simulink model "rpi_i2c_send"  (R2014a)
settings: Solver=FixedStepDiscrete  StartTime=0.0  StopTime=inf  RelTol=1e-3
libraries: embdlinuxlib x3, dspindex x2, visionstatistics x1, visiontextngfix x1, visionanalysis x1
settings Model: SimulationMode=external  ExtModeTrigDuration=100  Creator=mbelge  LastModifiedBy=planger
settings DataIOCC: SignalLoggingSaveFormat=ModelDataLogs
settings OptimizationCC: ExpressionDepthLimit=2147483647  OptimizeModelRefInitCode=on  LifeSpan=1
settings DebuggingCC: UnderspecifiedInitializationDetection=Classic  SolverPrmCheckMsg=none  FcnCallInpInsideContextMsg=EnableAllAsWarning  StateNameClashWarn=warning
settings HardwareCC: ProdLargestAtomicInteger=Long  ProdLargestAtomicFloat=Double  ProdEndianess=LittleEndian  ProdHWDeviceType=ARM Compatible->ARM Cortex
settings RTWCC: SystemTargetFile=realtime.tlc  GenerateMakefile=off  TemplateMakefile=realtime.tmf  Description=Real-Time Toolbox  RTWVerbose=off  ProcessScript=realtime_make_rtw_hook
settings CodeAppCC: CustomSymbolStrType=$N$R$M  InternalIdentifier=Classic
settings STFCustomTargetCC: TargetLibSuffix=.a  GenerateSampleERTMain=on  ConcurrentExecutionCompliant=off  GeneratePreprocessorConditionals=Use local settings  ERTCustomFileBanners=on  SupportNonInlinedSFcns=off  SupportVariableSizeSignals=on  MATLABClassNameForMDSCustomization=Simulink.SoftwareTarget.ERTCustomization  GRTInterface=off  SystemTargetFile=realtime.tlc
settings ERTTargetCC: CombineOutputUpdateFcns=off  SupportContinuousTime=on  SupportVariableSizeSignals=on  ExtMode=on  ExtModeMexArgs='plpi-wifi' 0 17725  ERTSrcFileBannerTemplate=realtime_code_template.cgt  ERTHdrFileBannerTemplate=realtime_code_template.cgt  ERTDataSrcFileTemplate=realtime_code_template.cgt  ERTDataHdrFileTemplate=realtime_code_template.cgt  ERTCustomFileTemplate=realtime_file_process.tlc

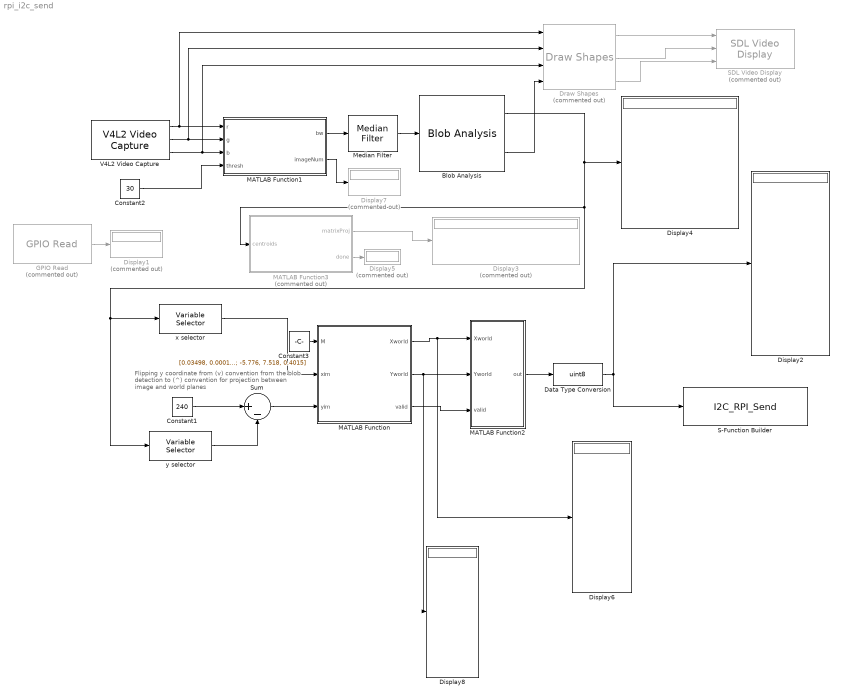
== system rpi_i2c_send ==
  note: Flipping y coordinate from (v) convention from
      | the blob detection to (^) convention for projection
      | between image and world planes
  Blob Analysis : visionstatistics/Blob Analysis  Tag=vipblks_row_conv  area=off  centroid=on  bBox=on  majorAxis=off  minorAxis=off  angle=off  eccentricity=off  equivDiameterSq=off  extent=off  perimeter=off  maxBlobs=6  warnIfNumBlobsExceeded=off  isCount=off  useMinArea=on  minArea=25  useMaxArea=off  maxArea=intmax('uint32')  excludeBorderBlob=on  outDT=single  isOutVarDim=off  isFill=on  fillValues=-1  conn=8  isLabel=off  outputMode=Binary point scaling  outputWordLength=32  outputFracLength=16  firstCoeffMode=Binary point scaling  firstCoeffWordLength=16  firstCoeffFracLength=14  secondCoeffMode=Binary point scaling  secondCoeffWordLength=32  secondCoeffFracLength=16  accumMode=Binary point scaling  accumWordLength=32  accumFracLength=0  prodOutputMode=Binary point scaling  prodOutputWordLength=32  prodOutputFracLength=16  roundingMode=Floor  overflowMode=off
  Constant1 : Constant  Value=240  OutDataTypeStr=single
  Constant2 : Constant  Value=30  OutDataTypeStr=single
  Constant3 : Constant  Value=[0.03498, 0.0001508, -4.339e-5; 0.001215, 0.01909, -0.001534; -5.776, 7.518, 0.4015]  VectorParams1D=off  OutDataTypeStr=single
  Data Type Conversion : DataTypeConversion  OutDataTypeStr=uint8
  Display{1,3,5,7} (4 alike) : Display  Commented=on
  Display{2,4,6,8} (4 alike) : Display
  Draw Shapes : visiontextngfix/Draw Shapes  Commented=on  shape=Rectangles  fill=off  lineWidth=1  fillClrSource=Specify via dialog  display=User-specified value  intensity=200  color=[0 0 0]  opacity=0.6  viewport=Entire image  antialiasing=off  inType=Obsolete  imagePorts=Separate color signals  prodOutputMode=Binary point scaling  prodOutputWordLength=32  prodOutputFracLength=14  memoryMode=Specify word length  memoryWordLength=16  memoryFracLength=15  roundingMode=Floor  overflowMode=off
  GPIO Read : embdlinuxlib/GPIO Read  Commented=on  board=Model B Rev2  gpio=4  internalResistor=Off  sampleTime=0.1  direction=Input  blockPlatform=Raspberry Pi
  MATLAB Function : MATLAB Function  TreatAsAtomicUnit=on
  MATLAB Function1 : MATLAB Function  TreatAsAtomicUnit=on
  MATLAB Function2 : MATLAB Function  TreatAsAtomicUnit=on
  MATLAB Function3 : MATLAB Function  Commented=on  TreatAsAtomicUnit=on
  Median Filter : visionanalysis/Median Filter  nghbood=[3 3]  outSize=Same as input port I  padType=Constant  padSrc=Specify via dialog  padVal=0  roundingMode=Floor  overflowMode=off
  S-Function Builder : S-Function  InitFcn=try, set_param(gcb,'FunctionName','I2C_RPI_Send'), end  FunctionName=I2C_RPI_Send  SFunctionModules=I2C_RPI_Send_wrapper  EnableBusSupport=off  mask(S-Function Builder){}
      mask help: Simulink:masks:SFunctionBuilder_MD
      mask init:
      | val = [[.9  0.75 0.75 1 1 .9 .9 1]',[1 1 0.75 0.75 .9 .9 1 .9]'];try , sys = get_param(gcb,'SfunBuilderFcnName');if isempty(sys), sys = get_param(gcb,'FunctionName'); end,catch, sys = get_param(gcb,'FunctionName'); end
      settings: CopyFcn=set_param(gcbh,'LinkStatus','none')  PreSaveFcn=try, set_param(gcb,'FunctionName','I2C_RPI_Send'), end  OpenFcn=sfunctionwizard(gcbh)
      mask Display: plot(val(:,1),val(:,2)),disp(sys), port_label('input',1,'Send')
  SDL Video Display : embdlinuxlib/SDL Video Display  Commented=on  pixelFormat=RGB  pixelOrder=Planar  rowMajor=on  blockPlatform=Raspberry Pi
  Sum : Sum  Inputs=|+-
  V4L2 Video Capture : embdlinuxlib/V4L2 Video Capture  m_devName='/dev/video0'  roi=[0, 0, 640, 480]  imSizeSelection=320x240  imSize=[640, 480]  pixelFormat=RGB  pixelOrder=Planar  sampleTime=1/10  simOutput=Colorbars  blockPlatform=Raspberry Pi
  x selector : dspindex/Variable Selector  NumInputs=1  rowsOrCols=Columns  IdxMode=Fixed  Elements=2  ZerOneIdxMode=One-based  errmode=Generate Error  FillMode=on  FillValues=0
  y selector : dspindex/Variable Selector  NumInputs=1  rowsOrCols=Columns  IdxMode=Fixed  Elements=1  ZerOneIdxMode=One-based  errmode=Generate Error  FillMode=on  FillValues=0
  wires:
  Data Type Conversion/1 -> Display2/1, S-Function Builder/1
  Blob Analysis/1 -> x selector/1, y selector/1, MATLAB Function3/1(centroids), Display4/1
  y selector/1 -> Sum/2
  Constant1/1 -> Sum/1
  Sum/1 -> MATLAB Function/3(yim)
  x selector/1 -> MATLAB Function/2(xim)
  V4L2 Video Capture/3 -> MATLAB Function1/3(b), Draw Shapes/3
  V4L2 Video Capture/2 -> MATLAB Function1/2(g), Draw Shapes/2
  V4L2 Video Capture/1 -> MATLAB Function1/1(r), Draw Shapes/1
  Draw Shapes/3 -> SDL Video Display/3
  Draw Shapes/1 -> SDL Video Display/1
  Draw Shapes/2 -> SDL Video Display/2
  Constant2/1 -> MATLAB Function1/4(thresh)
  Median Filter/1 -> Blob Analysis/1
  MATLAB Function1/1(bw) -> Median Filter/1
  Blob Analysis/2 -> Draw Shapes/4
  MATLAB Function/2(Yworld) -> Display8/1, MATLAB Function2/2(Yworld)
  MATLAB Function2/1(out) -> Data Type Conversion/1
  MATLAB Function/1(Xworld) -> Display6/1, MATLAB Function2/1(Xworld)
  MATLAB Function1/2(imageNum) -> Display7/1
  MATLAB Function/3(valid) -> MATLAB Function2/3(valid)
  MATLAB Function3/1(matrixProj) -> Display3/1
  GPIO Read/1 -> Display1/1
  MATLAB Function3/2(done) -> Display5/1
  Constant3/1 -> MATLAB Function/1(M)

== matlab function rpi_i2c_send/MATLAB Function1 ==
  data: r input; bw output; g input; b input; thresh input; imageNum output
function [bw, imageNum] = greenDetect(r, g, b, thresh)
%#codegen

persistent counter
if isempty(counter)
    counter = 1;
end
    

justGreen = single(g) - single(r)/2 - single(b)/2;

bw = justGreen > thresh;

counter = counter + 1;
imageNum = counter;

== matlab function rpi_i2c_send/MATLAB Function ==
  data: M input; Xworld output; xim input; yim input; Yworld output; valid output
function [Xworld, Yworld, valid] = image2world(M, xim, yim)
%#codegen

% Inputs: xim = [nx1] vector of x-coordinate in image plane
%         yim = [nx1] vector of y-coordinate in image plane
%         
%         For the image coordinates, origin is bottom left, convention:
%         x (>), y(^)
%
% Outputs: Xworld = [nx1] vector of x-coordinates in world plane
%          Yworld = [nx1] vector of y-coordinates in world plane
%          
%          For the world coordinates, robot at (X,Y) = (0,0)
%

% if size(xim, 2) > size(xim, 1)
%     xim = xim' ;
% end
% 
% if size(yim, 2) > size(yim, 1)
%     yim = yim' ;
% end
    
% [Xworld,Yworld] = transformPointsInverse(t_world2im, xim, yim) ;
% transformPointsInverse does not support codegen, but can get code from
% its class projective2d.

% M = inv( t_world2im );
u = M(1,1).*xim + M(2,1).*yim + M(3,1);
v = M(1,2).*xim + M(2,2).*yim + M(3,2);
w = M(1,3).*xim + M(2,3).*yim + M(3,3);

Xworld = u./w ;
Yworld = v./w ;

% limite the minimum Yworld to 0
%Yworld = max([Yworld, zeros(size(Yworld))],[],2) ;

valid = ~(xim == -1);

== matlab function rpi_i2c_send/MATLAB Function2 ==
  data: Xworld input; out output; Yworld input; valid input
function out  = fcn(Xworld, Yworld, valid)
%#codegen

angles = atan2d(Yworld , Xworld);
distances = sqrt(Xworld.^2 + Yworld.^2); % already in cm

angles = angles .* valid;
distances = distances .* valid;
out = [ distances', angles'];

== matlab function rpi_i2c_send/MATLAB Function3 ==
  data: centroids input; matrixProj output; done output
function [matrixProj, done] = calib(centroids)
%#codegen
centroids = single(centroids);
matrixProj = single( [-0.0101    0.0008    0.0000;
                      -0.0002    0.0015    0.0005;
                       1.7075   -3.4207   -0.1261] );

% matrixProj = single( zeros(3,3) );

persistent calibrated calibCounter
if isempty( calibrated )
    calibrated = false;
    calibCounter = single(1);
end

if ~calibrated
    % image points, pixel coordinates, assuming resolution of the camera =
    % [240x320]
    % (>) x (^) y
    numPointsToUse = 4;
    numrows = single(240) ;
    yi = numrows - centroids(1:numPointsToUse, 1);  % from (v) to (^)
    xi = centroids(1:numPointsToUse, 2); % (>)
    
    % match the points to the 4 in the world
    topPtsInds = yi > mean(yi) ;
    bottomPtsInds = ~topPtsInds;
    leftPtsInds = xi < mean(xi) ;
    rightPtsInds = ~leftPtsInds ;
    
    
    imagePoints = [xi(topPtsInds & leftPtsInds), yi(topPtsInds & leftPtsInds) ;             % top left
                   xi(topPtsInds & rightPtsInds), yi(topPtsInds & rightPtsInds) ;           % top right
                   xi(bottomPtsInds & leftPtsInds), yi(bottomPtsInds & leftPtsInds) ;       % bottom left
                   xi( bottomPtsInds & rightPtsInds), yi(bottomPtsInds & rightPtsInds)];    % bottom right
               
    
    % world points (for four points on corners of A3 paper)
    %     1      2
    %   3          4
    % + change of origin
    Xw = [0,    0.297,  0,  0.297  ] - 0.297/2; % (>)
    Yw = [0.42, 0.42,   0,  0] + 0.42; % (^)
    worldPoints = [Xw', Yw'] * 100; % in cm
    
    [worldPoints,normMatrix_world] = myNormalizeControlPoints(worldPoints);
    [imagePoints,normMatrix_image] = myNormalizeControlPoints(imagePoints);

    minRequiredNonCollinearPairs = 4;
    M = size(imagePoints,1);
    x = imagePoints(:,1);
    y = imagePoints(:,2);
    vec_1 = ones(M,1);
    vec_0 = zeros(M,1);
    u = worldPoints(:,1);
    v = worldPoints(:,2);
    
    U = [u; v];
    
    X = [x      y      vec_1  vec_0  vec_0  vec_0  -u.*x  -u.*y;
        vec_0  vec_0  vec_0  x      y      vec_1  -v.*x  -v.*y  ];
    
    Tvec = zeros(9,1,'single');
    % We know that X * Tvec = U
    if rank(X) >= 2*minRequiredNonCollinearPairs
        Tvec(1:8) = X \ U;
    else
        error('calib failed')
    end
    
    % We assumed I = 1;
    Tvec(9) = single(1);
    
    Tinv = reshape(Tvec,3,3);
    Tinv = normMatrix_image \ (Tinv * normMatrix_world);
    
    T = inv(Tinv);
    T = T ./ T(3,3);
    matrixProj = single( inv( T ) ) % image to world projection
    calibCounter = calibCounter + single(1);
    
    calibrated = calibCounter >= single(1000);
    %save matrixCalib matrixProj
    done = calibrated;
else
    done = false;
end
